simulink model "FMS"  (R2021b)
settings: Solver=VariableStepAuto  StartTime=0.0  StopTime=10.0  RelTol=1e-3
settings Model: Creator=lhubl  LastModifiedBy=camil

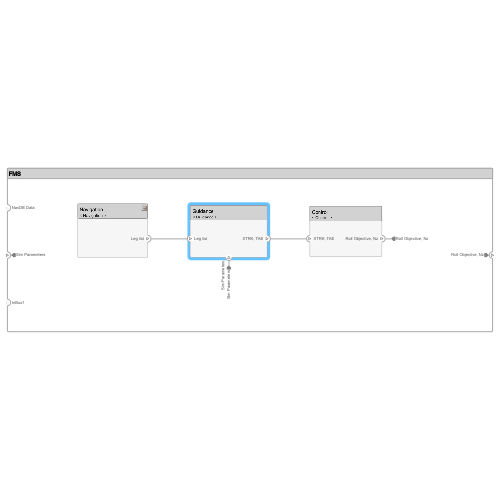
[thumbnail: Simulink's stored preview of the top-level diagram]
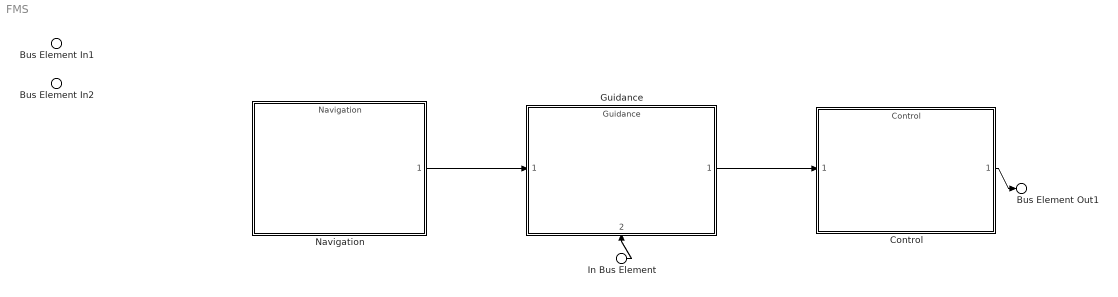
== system FMS ==
  Bus Element In1 : Inport  RequirementInfo={} %GIDa_306aa024_e9f3_4077_a4fc_4c981dd7b9aa  PortName=NavDB Data
  In Bus Element : Inport  Port=2  PortName=Sim Parameters
  Bus Element In2 : Inport  RequirementInfo={} %GIDa_8f0b7339_79c7_4f56_9401_39d029561790  Port=3  PortName=InBus1
  Control : ModelReference  ModelNameDialog=Control  SimulationMode=Normal  ModelReferenceVersion=1.1
      settings: PortSchema="{\"entries\":[{\"content\":{\"headerSize\":38,\"margin\":15,\"minimumSpacing\":25,\"sides\":[{\"content\":{\"connectorIds\":[\"In1\"]},\"type\":\"ConnectorPlacement.EquallySpacedRectSide\",\"uuid\":\"f0697a98-65c4-48b6-9148-6d90a1a908b8\"},{\"content\":{\"connectorIds\":[\"Out1\"],\"side\":\"RIGHT\"},\"type\":\"ConnectorPlacement.EquallySpacedRectSide\",\"uuid\":\"c62a382e-4014-433d-b035-2a8a1906ece2\"},{\"content\":{\"connectorIds\":[],\"side\":\"TOP\"},\"type\":\"ConnectorPlacement.EquallySpacedRectSide\",\"uuid\":\"02cc979b-05b8-4cbd-9662-94fbd431603b\"}]},\"type\":\"ConnectorPlacement.EquallySpacedConnector\",\"uuid\":\"1201885f-d543-4e5c-981e-efbc8a5dca28\"}],\"packageUris\":[\"http://schema.mathworks.com/mf0/Connector/R2020b\"],\"version\":\"1.0\"}"
  "Guidance " : ModelReference  ModelNameDialog=Guidance  SimulationMode=Normal  ModelReferenceVersion=1.2
      settings: PortSchema="{\"entries\":[{\"content\":{\"headerSize\":38,\"margin\":15,\"minimumSpacing\":25,\"sides\":[{\"content\":{\"connectorIds\":[\"In1\"]},\"type\":\"ConnectorPlacement.EquallySpacedRectSide\",\"uuid\":\"f0697a98-65c4-48b6-9148-6d90a1a908b8\"},{\"content\":{\"connectorIds\":[\"Out1\"],\"side\":\"RIGHT\"},\"type\":\"ConnectorPlacement.EquallySpacedRectSide\",\"uuid\":\"c62a382e-4014-433d-b035-2a8a1906ece2\"},{\"content\":{\"connectorIds\":[],\"side\":\"TOP\"},\"type\":\"ConnectorPlacement.EquallySpacedRectSide\",\"uuid\":\"02cc979b-05b8-4cbd-9662-94fbd431603b\"},{\"content\":{\"connectorIds\":[\"In2\"],\"side\":\"BOTTOM\"},\"type\":\"ConnectorPlacement.EquallySpacedRectSide\",\"uuid\":\"5bdaab2e-938c-4b83-b2da-198f1945ee00\"}]},\"type\":\"ConnectorPlacement.EquallySpacedConnector\",\"uuid\":\"1201885f-d543-4e5c-981e-efbc8a5dca28\"}],\"packageUris\":[\"http://schema.mathworks.com/mf0/Connector/R2020b\"],\"version\":\"1.0\"}"
  Navigation : ModelReference  ModelNameDialog=Navigation  SimulationMode=Normal  ModelReferenceVersion=1.1
      settings: PortSchema="{\"entries\":[{\"content\":{\"headerSize\":38,\"margin\":15,\"minimumSpacing\":25,\"sides\":[{\"content\":{\"connectorIds\":[]},\"type\":\"ConnectorPlacement.EquallySpacedRectSide\",\"uuid\":\"f0697a98-65c4-48b6-9148-6d90a1a908b8\"},{\"content\":{\"connectorIds\":[\"Out1\"],\"side\":\"RIGHT\"},\"type\":\"ConnectorPlacement.EquallySpacedRectSide\",\"uuid\":\"c62a382e-4014-433d-b035-2a8a1906ece2\"},{\"content\":{\"connectorIds\":[],\"side\":\"TOP\"},\"type\":\"ConnectorPlacement.EquallySpacedRectSide\",\"uuid\":\"02cc979b-05b8-4cbd-9662-94fbd431603b\"}]},\"type\":\"ConnectorPlacement.EquallySpacedConnector\",\"uuid\":\"1201885f-d543-4e5c-981e-efbc8a5dca28\"}],\"packageUris\":[\"http://schema.mathworks.com/mf0/Connector/R2020b\"],\"version\":\"1.0\"}"
  Bus Element Out1 : Outport  RequirementInfo={} %GIDa_68c6b491_cecf_42b1_babe_de608741fe37  PortName=Roll Objective, Nz
  wires:
  Navigation/1 -> "Guidance "/1
  "Guidance "/1 -> Control/1
  Control/1 -> Bus Element Out1/1
  In Bus Element/1 -> "Guidance "/2
